simulink model "ROV_Simulation_openloop_ver2"  (R2023a)
settings: Solver=ode15s  StartTime=0.0  StopTime=Sim.ts  FixedStep=0.01  MaxStep=0.01  MinStep=0.0001  RelTol=1e-3
undefined symbols (not defined in the file): ext, hyd, ics, phy, rb, thrust, VC
libraries: simulink_extras x3, simulink x1
settings Model: Creator=dmmavani  LastModifiedBy=dmmavani
settings SolverCC: ConcurrentTasks=on  PositivePriorityOrder=on  AutoInsertRateTranBlk=on
settings DataIOCC: InspectSignalLogs=on
settings OptimizationCC: BlockReduction=off  DefaultParameterBehavior=Inlined  EnhancedBackFolding=on  PassReuseOutputArgsAs=Individual arguments  ZeroExternalMemoryAtStartup=off  ZeroInternalMemoryAtStartup=off  OptimizeBlockOrder=speed  DifferentSizesBufferReuse=on  OptimizationCustomize=off  EfficientTunableParamExpr=on
settings DebuggingCC: TasksWithSamePriorityMsg=none  ParameterTunabilityLossMsg=error
settings HardwareCC: ProdBitPerLong=64  ProdLongLongMode=on  ProdHWDeviceType=Intel->x86-64 (Linux 64)
settings SFSimCC: MATLABDynamicMemAlloc=off
settings RTWCC: Description=Embedded Coder  SystemTargetFile=ert.tlc  GenCodeOnly=on  TemplateMakefile=ert_default_tmf  Toolchain=Simulink Real-Time Toolchain  BuildConfiguration=Faster Runs  CodeExecutionProfiling=on  TargetLang=C++
settings CodeAppCC: ForceParamTrailComments=on  IgnoreCustomStorageClasses=off  OperatorAnnotations=on  SimulinkDataObjDesc=on  SFDataObjDesc=on  InsertBlockDesc=on
settings ERTTargetCC: TargetLangStandard=C++03 (ISO)  GenerateSampleERTMain=on  CodeInterfacePackaging=C++ class  InlinedParameterPlacement=NonHierarchical  RootIOFormat=Structure reference  ERTCustomFileTemplate=example_file_process.tlc

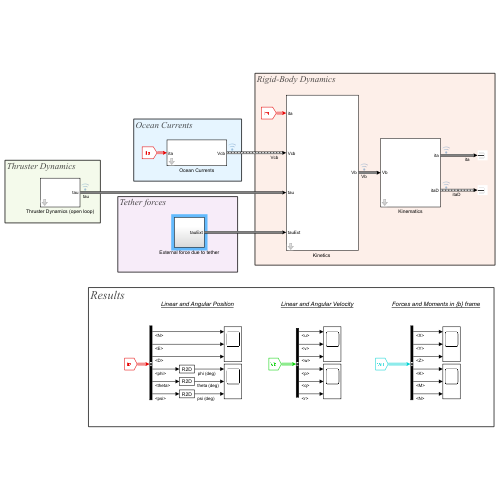
[thumbnail: Simulink's stored preview of the top-level diagram]
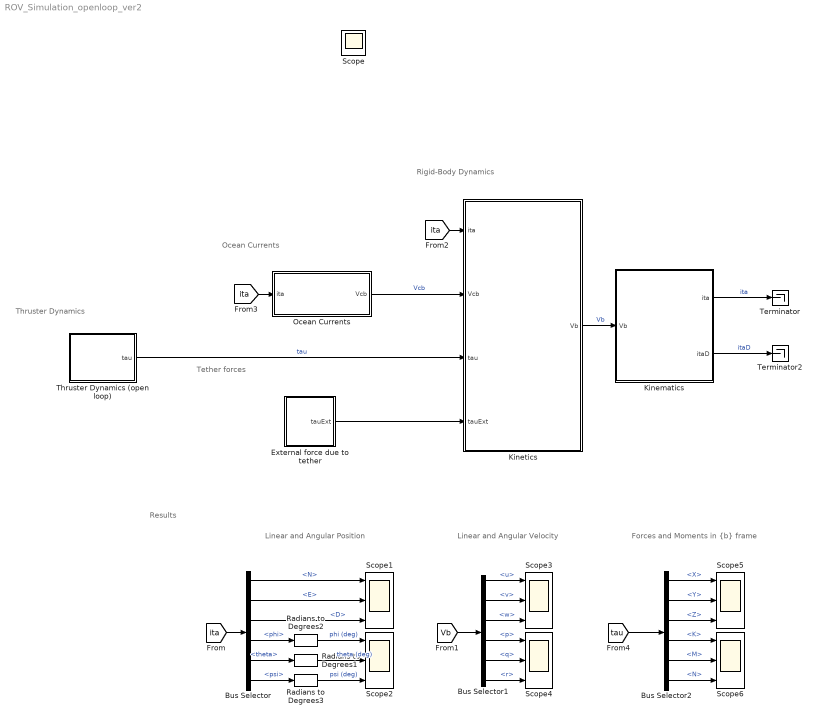
== system ROV_Simulation_openloop_ver2 ==
  note: Results
  note: Linear and Angular Position
  note: Tether forces
  note: Thruster Dynamics
  note: Ocean Currents
  note: Rigid-Body Dynamics
  note: Linear and Angular Velocity
  note: Forces and Moments in {b} frame
  Bus Selector : BusSelector  OutputSignals=N,E,D,phi,theta,psi
  Bus Selector1 : BusSelector  OutputSignals=u,v,w,p,q,r
  Bus Selector2 : BusSelector  OutputSignals=X,Y,Z,K,M,N
  External force due to tether : Subsystem
  Kinematics : Subsystem  mask{Parameter7=|, North=ics.ita.N, East=ics.ita.E, Down=ics.ita.D, Roll=ics.ita.phi, Pitch=ics.ita.theta, InitialCondition=ics.ita.psi}
      mask Parameter7=|
      | Kinematics block is used to transform velocities from BODY to
      | NED frame.
      |
      | itaD = J(euler) * Vb    ( Velocities in NED frame)
      | J(euler) = Transformation Matrix (function of euler angles)
      | Vb = Velocities in BODY frame.
      mask prompts: North "N :"; East "E :"; Down "D :"; Roll "Roll :"; Pitch "Pitch :"; InitialCondition "Yaw :"
      mask TypeOptions North: Integrator/InitialCondition
      mask TypeOptions East: Integrator1/InitialCondition
      mask TypeOptions Down: Integrator3/InitialCondition
      mask TypeOptions Roll: Integrator4/InitialCondition
      mask TypeOptions Pitch: Integrator5/InitialCondition
      mask TypeOptions InitialCondition: Integrator6/InitialCondition
      mask DialogControl Container4 Prompt: Description
      mask DialogControl Container1 Prompt: Initial Conditions for position and orientation in NED frame
      mask DialogControl Container2 Prompt: Position (meters)
      mask DialogControl Container3 Prompt: Orientation (rad)
  "Kinetics " : Subsystem  mask{Parameter7=|, u_b=ics.vb.u, v_b=ics.vb.v, w_b=ics.vb.w, p_b=ics.vb.p, q_b=ics.vb.q, r_b=ics.vb.r}
      mask Parameter7=|
      | Kinetics block is used to solve the 6DOF equations of motion
      | of a ROV in BODY frame.
      | Block outputs V_b (Velocities in BODY frame).
      mask prompts: u_b "u_b :"; v_b "v_b :"; w_b "w_b :"; p_b "p_b :"; q_b "q_b :"; r_b "r_b :"
      mask TypeOptions u_b: Integrator/InitialCondition
      mask TypeOptions v_b: Integrator1/InitialCondition
      mask TypeOptions w_b: Integrator2/InitialCondition
      mask TypeOptions p_b: Integrator3/InitialCondition
      mask TypeOptions q_b: Integrator4/InitialCondition
      mask TypeOptions r_b: Integrator5/InitialCondition
      mask DialogControl Container4 Prompt: Description
      mask DialogControl InitialCondition Prompt: Initial conditions for velocity of body in {b} frame
      mask DialogControl Container2 Prompt: Linear Velocity  (m/s)
      mask DialogControl Container3 Prompt: Angular Velocity (rad/s)
  Ocean Currents : Subsystem  mask{Parameter1=|, Value=VC}
      mask Parameter1=|
      | If the value is equal to 1 then ocean currents is ON.
      | if the value is equal to 0 then ocean currents is OFF.
      mask prompts: Value "Ocean currents (On/Off):"
      mask TypeOptions Value: Constant1/Value
      mask DialogControl Container2 Prompt: Description
  Radians to Degrees1 : simulink_extras/Transformations/Radians to Degrees
  Radians to Degrees2 : simulink_extras/Transformations/Radians to Degrees
  Radians to Degrees3 : simulink_extras/Transformations/Radians to Degrees
  Scope{1..6} (6 alike) : Scope  NumInputPorts=3
  Terminator : Terminator
  Terminator2 : Terminator
  Thruster Dynamics (open loop) : Subsystem  mask{Parameter2=|, Value=1}
      mask Parameter2=|
      | Step input    (Input type = 1)
      | Impulse input (Input type = 0)
      mask prompts: Value "Input type:"
      mask TypeOptions Value: Constant/Value
      mask DialogControl DescGroupVar Prompt: Description
  Scope : Scope
  wires:
  Ocean Currents/1(Vcb) -> "Kinetics "/2(Vcb)  "Vcb"
  [ita] -> Bus Selector/1
  Bus Selector/1 -> Scope1/1  "<N>"
  Bus Selector/2 -> Scope1/2  "<E>"
  Bus Selector/3 -> Scope1/3  "<D>"
  Bus Selector/4 -> Radians to Degrees2/1  "<phi>"
  Radians to Degrees2/1 -> Scope2/1  "phi (deg)"
  Bus Selector/5 -> Radians to Degrees1/1  "<theta>"
  Bus Selector/6 -> Radians to Degrees3/1  "<psi>"
  [Vb] -> Bus Selector1/1
  Bus Selector1/1 -> Scope3/1  "<u>"
  Bus Selector1/2 -> Scope3/2  "<v>"
  Bus Selector1/3 -> Scope3/3  "<w>"
  Bus Selector1/4 -> Scope4/1  "<p>"
  Bus Selector1/5 -> Scope4/2  "<q>"
  Bus Selector1/6 -> Scope4/3  "<r>"
  Kinematics/1(ita) -> Terminator/1  "ita"
  [ita] -> Ocean Currents/1(ita)
  Thruster Dynamics (open loop)/1(tau) -> "Kinetics "/3(tau)  "tau"
  "Kinetics "/1(Vb) -> Kinematics/1(Vb)  "Vb"
  Kinematics/2(itaD) -> Terminator2/1  "itaD"
  [ita] -> "Kinetics "/1(ita)
  [tau] -> Bus Selector2/1
  Bus Selector2/1 -> Scope5/1  "<X>"
  Bus Selector2/2 -> Scope5/2  "<Y>"
  Bus Selector2/3 -> Scope5/3  "<Z>"
  Bus Selector2/4 -> Scope6/1  "<K>"
  Bus Selector2/5 -> Scope6/2  "<M>"
  Bus Selector2/6 -> Scope6/3  "<N>"
  Radians to Degrees1/1 -> Scope2/2  "theta (deg)"
  Radians to Degrees3/1 -> Scope2/3  "psi (deg)"
  External force due to tether/1(tauExt) -> "Kinetics "/4(tauExt)

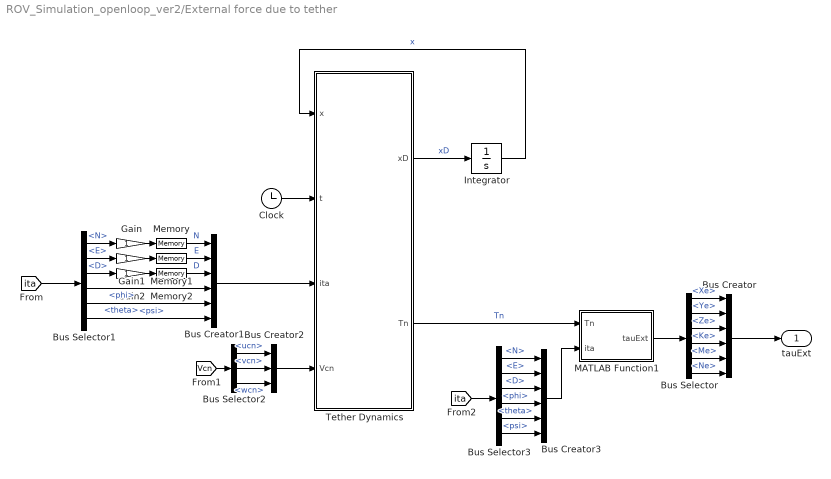
== system ROV_Simulation_openloop_ver2/External force due to tether ==
  Bus Creator : BusCreator  Inputs=6  OutDataTypeStr=Bus: tauExt
  Bus Creator1 : BusCreator  Inputs=6  OutDataTypeStr=Bus: ita
  Bus Creator2 : BusCreator  Inputs=3  OutDataTypeStr=Bus: Vcn
  Bus Creator3 : BusCreator  Inputs=6  OutDataTypeStr=Bus: ita
  Bus Selector : BusSelector  OutputSignals=Xe,Ye,Ze,Ke,Me,Ne
  Bus Selector1 : BusSelector  OutputSignals=N,E,D,phi,theta,psi
  Bus Selector2 : BusSelector  OutputSignals=ucn,vcn,wcn
  Bus Selector3 : BusSelector  OutputSignals=N,E,D,phi,theta,psi
  Clock : Clock
  Gain : Gain
  Gain1 : Gain
  Gain2 : Gain
  Integrator : Integrator  InitialCondition=ics.tether.xstate
  MATLAB Function1 : MATLAB Function  TreatAsAtomicUnit=on
  Memory : Memory  InitialCondition=ics.ita.N
  Memory1 : Memory  InitialCondition=ics.ita.E
  Memory2 : Memory  InitialCondition=ics.ita.D
  Tether Dynamics : MATLAB Function  TreatAsAtomicUnit=on
  tauExt : Outport  OutDataTypeStr=Bus: tauExt
  wires:
  Gain1/1 -> Memory1/1
  Gain2/1 -> Memory2/1
  Bus Selector1/6 -> Bus Creator1/6  "<psi>"
  Memory2/1 -> Bus Creator1/3  "D"
  Memory1/1 -> Bus Creator1/2  "E"
  Bus Creator2/1 -> Tether Dynamics/4(Vcn)
  Tether Dynamics/1(xD) -> Integrator/1  "xD"
  Gain/1 -> Memory/1
  Bus Creator3/1 -> MATLAB Function1/2(ita)
  Bus Selector3/5 -> Bus Creator3/5  "<theta>"
  Bus Selector1/1 -> Gain/1  "<N>"
  Bus Selector2/1 -> Bus Creator2/1  "<ucn>"
  [Vcn] -> Bus Selector2/1
  Clock/1 -> Tether Dynamics/2(t)
  Bus Selector3/4 -> Bus Creator3/4  "<phi>"
  Bus Selector3/1 -> Bus Creator3/1  "<N>"
  Integrator/1 -> Tether Dynamics/1(x)  "x"
  MATLAB Function1/1(tauExt) -> Bus Selector/1
  Bus Selector3/2 -> Bus Creator3/2  "<E>"
  [ita] -> Bus Selector1/1
  Memory/1 -> Bus Creator1/1  "N"
  Bus Selector1/5 -> Bus Creator1/5  "<theta>"
  [ita] -> Bus Selector3/1
  Bus Selector1/4 -> Bus Creator1/4  "<phi>"
  Bus Selector3/3 -> Bus Creator3/3  "<D>"
  Bus Selector1/2 -> Gain1/1  "<E>"
  Tether Dynamics/2(Tn) -> MATLAB Function1/1(Tn)  "Tn"
  Bus Selector/6 -> Bus Creator/6  "<Ne>"
  Bus Selector1/3 -> Gain2/1  "<D>"
  Bus Creator1/1 -> Tether Dynamics/3(ita)
  Bus Selector/4 -> Bus Creator/4  "<Ke>"
  Bus Selector/5 -> Bus Creator/5  "<Me>"
  Bus Selector/3 -> Bus Creator/3  "<Ze>"
  Bus Selector/2 -> Bus Creator/2  "<Ye>"
  Bus Selector2/2 -> Bus Creator2/2  "<vcn>"
  Bus Creator/1 -> tauExt/1
  Bus Selector2/3 -> Bus Creator2/3  "<wcn>"
  Bus Selector/1 -> Bus Creator/1  "<Xe>"
  Bus Selector3/6 -> Bus Creator3/6  "<psi>"

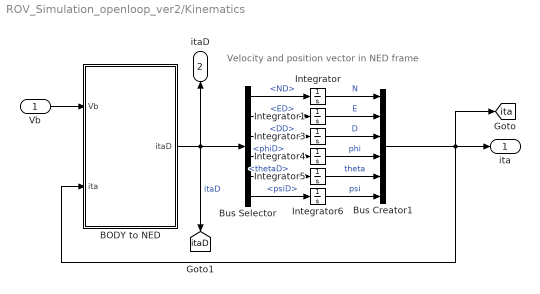
== system ROV_Simulation_openloop_ver2/Kinematics ==
  note: Velocity and position vector in
      |  NED frame
  Vb : Inport  OutDataTypeStr=Bus: Vb
  " BODY to NED" : MATLAB Function  TreatAsAtomicUnit=on
  Bus Creator1 : BusCreator  Inputs=6  OutDataTypeStr=Bus: ita
  Bus Selector : BusSelector  OutputSignals=ND,ED,DD,phiD,thetaD,psiD
  Integrator : Integrator  InitialCondition=North  LowerSaturationLimit=ics.N
  Integrator1 : Integrator  InitialCondition=East  LowerSaturationLimit=ics.E
  Integrator3 : Integrator  InitialCondition=Down  LowerSaturationLimit=ics.D
  Integrator4 : Integrator  InitialCondition=Roll  LowerSaturationLimit=ics.phi
  Integrator5 : Integrator  InitialCondition=Pitch  LowerSaturationLimit=ics.theta
  Integrator6 : Integrator  InitialCondition=InitialCondition  LowerSaturationLimit=ics.psi
  ita : Outport  OutDataTypeStr=Bus: ita
  itaD : Outport  Port=2  OutDataTypeStr=Bus: itaD
  tag scope: ita=global, itaD=global
  wires:
  " BODY to NED"/1(itaD) -> Bus Selector/1, [itaD], itaD/1  "itaD"
  Bus Creator1/1 -> [ita], ita/1, " BODY to NED"/2(ita)
  Bus Selector/1 -> Integrator/1  "<ND>"
  Bus Selector/2 -> Integrator1/1  "<ED>"
  Bus Selector/6 -> Integrator6/1  "<psiD>"
  Bus Selector/5 -> Integrator5/1  "<thetaD>"
  Bus Selector/3 -> Integrator3/1  "<DD>"
  Bus Selector/4 -> Integrator4/1  "<phiD>"
  Integrator/1 -> Bus Creator1/1  "N"
  Integrator1/1 -> Bus Creator1/2  "E"
  Integrator3/1 -> Bus Creator1/3  "D"
  Integrator4/1 -> Bus Creator1/4  "phi"
  Integrator5/1 -> Bus Creator1/5  "theta"
  Integrator6/1 -> Bus Creator1/6  "psi"
  Vb/1 -> " BODY to NED"/1(Vb)

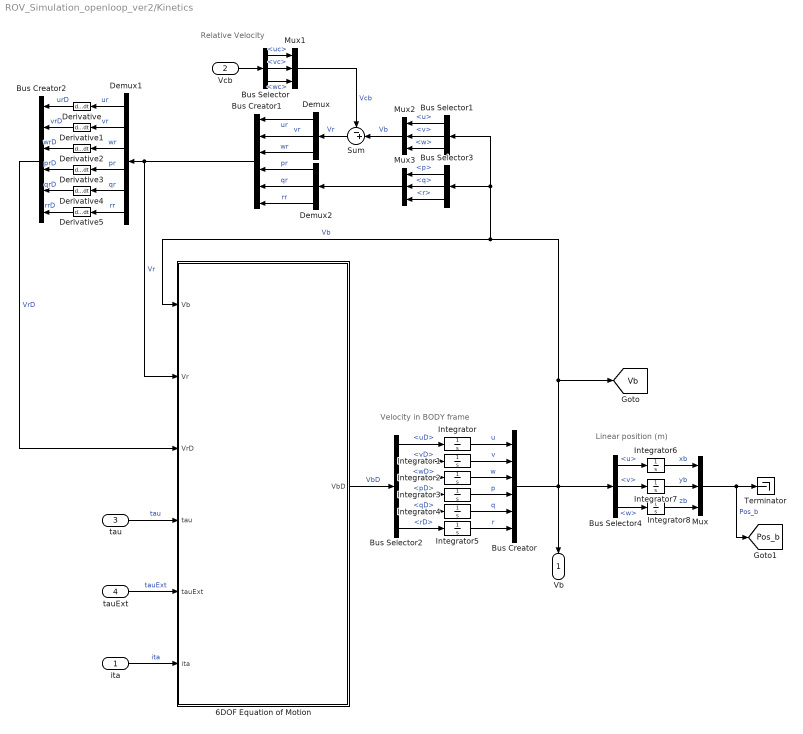
== system ROV_Simulation_openloop_ver2/Kinetics  ==
  note: Linear position (m)
  note: Velocity in BODY frame
  note: Relative Velocity
  ita : Inport  OutDataTypeStr=Bus: ita
  Vcb : Inport  Port=2  OutDataTypeStr=Bus: Vcb
  tau : Inport  Port=3  OutDataTypeStr=Bus: tau
  tauExt : Inport  Port=4  OutDataTypeStr=Bus: tauExt
  "6DOF Equation of Motion " : MATLAB Function  TreatAsAtomicUnit=on
  Bus Creator : BusCreator  Inputs=6  OutDataTypeStr=Bus: Vb
  Bus Creator1 : BusCreator  Inputs=6  OutDataTypeStr=Bus: Vr
  Bus Creator2 : BusCreator  Inputs=6  OutDataTypeStr=Bus: VrD
  Bus Selector : BusSelector  OutputSignals=uc,vc,wc
  Bus Selector1 : BusSelector  OutputSignals=u,v,w
  Bus Selector2 : BusSelector  OutputSignals=uD,vD,wD,pD,qD,rD
  Bus Selector3 : BusSelector  OutputSignals=p,q,r
  Bus Selector4 : BusSelector  OutputSignals=u,v,w
  Demux : Demux  Outputs=3
  Demux1 : Demux  Outputs=6
  Demux2 : Demux  Outputs=3
  Derivative{,1..5} (6 alike) : Derivative
  Integrator : Integrator  InitialCondition=u_b  UpperSaturationLimit=ics.sat.umax  LowerSaturationLimit=0
  Integrator1 : Integrator  InitialCondition=v_b  UpperSaturationLimit=ics.sat.vmax  LowerSaturationLimit=0
  Integrator2 : Integrator  InitialCondition=w_b  UpperSaturationLimit=ics.sat.wmax  LowerSaturationLimit=0
  Integrator3 : Integrator  InitialCondition=p_b  UpperSaturationLimit=ics.sat.pmax  LowerSaturationLimit=0
  Integrator4 : Integrator  InitialCondition=q_b  UpperSaturationLimit=ics.sat.qmax  LowerSaturationLimit=0
  Integrator5 : Integrator  InitialCondition=r_b  UpperSaturationLimit=ics.sat.rmax  LowerSaturationLimit=0
  Integrator6 : Integrator  LowerSaturationLimit=0
  Integrator7 : Integrator  LowerSaturationLimit=0
  Integrator8 : Integrator  LowerSaturationLimit=0
  Mux{,1..3} (4 alike) : Mux  Inputs=3
  Sum : Sum  Inputs=-+|
  Terminator : Terminator
  Vb : Outport  OutDataTypeStr=Bus: Vb
  tag scope: Pos_b=global, Vb=global
  wires:
  Mux1/1 -> Sum/1  "Vcb"
  Bus Selector1/1 -> Mux2/1  "<u>"
  Bus Selector1/2 -> Mux2/2  "<v>"
  Bus Selector1/3 -> Mux2/3  "<w>"
  Mux2/1 -> Sum/2  "Vb"
  Bus Creator/1 -> Bus Selector1/1, Bus Selector3/1, "6DOF Equation of Motion "/1(Vb), [Vb], Vb/1, Bus Selector4/1  "Vb"
  ita/1 -> "6DOF Equation of Motion "/6(ita)  "ita"
  tau/1 -> "6DOF Equation of Motion "/4(tau)  "tau"
  "6DOF Equation of Motion "/1(VbD) -> Bus Selector2/1  "VbD"
  Bus Selector2/1 -> Integrator/1  "<uD>"
  Bus Selector2/2 -> Integrator1/1  "<vD>"
  Bus Selector2/3 -> Integrator2/1  "<wD>"
  Bus Selector2/4 -> Integrator3/1  "<pD>"
  Bus Selector2/5 -> Integrator4/1  "<qD>"
  Bus Selector2/6 -> Integrator5/1  "<rD>"
  Vcb/1 -> Bus Selector/1
  Bus Selector/1 -> Mux1/1  "<uc>"
  Bus Selector/2 -> Mux1/2  "<vc>"
  Bus Selector/3 -> Mux1/3  "<wc>"
  Sum/1 -> Demux/1  "Vr"
  Demux/1 -> Bus Creator1/1  "ur"
  Demux/3 -> Bus Creator1/3  "wr"
  Mux3/1 -> Demux2/1
  Demux/2 -> Bus Creator1/2  "vr"
  Demux2/1 -> Bus Creator1/4  "pr"
  Demux2/2 -> Bus Creator1/5  "qr"
  Demux2/3 -> Bus Creator1/6  "rr"
  Integrator/1 -> Bus Creator/1  "u"
  Integrator1/1 -> Bus Creator/2  "v"
  Integrator2/1 -> Bus Creator/3  "w"
  Integrator3/1 -> Bus Creator/4  "p"
  Integrator4/1 -> Bus Creator/5  "q"
  Integrator5/1 -> Bus Creator/6  "r"
  Bus Selector3/2 -> Mux3/2  "<q>"
  Bus Selector3/3 -> Mux3/3  "<r>"
  Bus Selector3/1 -> Mux3/1  "<p>"
  Bus Selector4/1 -> Integrator6/1  "<u>"
  Bus Selector4/2 -> Integrator7/1  "<v>"
  Bus Selector4/3 -> Integrator8/1  "<w>"
  Integrator6/1 -> Mux/1  "xb"
  Integrator7/1 -> Mux/2  "yb"
  Integrator8/1 -> Mux/3  "zb"
  Mux/1 -> [Pos_b], Terminator/1  "Pos_b"
  Bus Creator1/1 -> Demux1/1, "6DOF Equation of Motion "/2(Vr)  "Vr"
  Demux1/1 -> Derivative/1  "ur"
  Derivative/1 -> Bus Creator2/1  "urD"
  Demux1/2 -> Derivative1/1  "vr"
  Derivative1/1 -> Bus Creator2/2  "vrD"
  Demux1/3 -> Derivative2/1  "wr"
  Derivative2/1 -> Bus Creator2/3  "wrD"
  Demux1/4 -> Derivative3/1  "pr"
  Derivative3/1 -> Bus Creator2/4  "prD"
  Demux1/5 -> Derivative4/1  "qr"
  Derivative4/1 -> Bus Creator2/5  "qrD"
  Demux1/6 -> Derivative5/1  "rr"
  Derivative5/1 -> Bus Creator2/6  "rrD"
  Bus Creator2/1 -> "6DOF Equation of Motion "/3(VrD)  "VrD"
  tauExt/1 -> "6DOF Equation of Motion "/5(tauExt)  "tauExt"

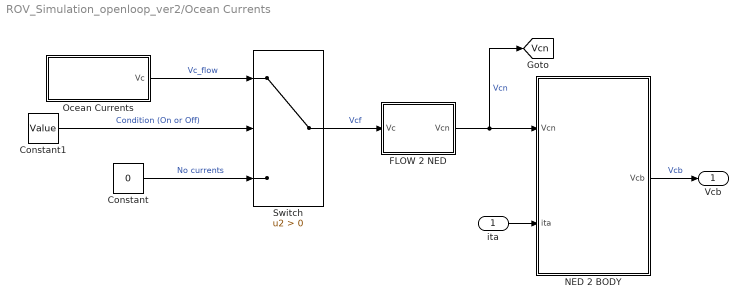
== system ROV_Simulation_openloop_ver2/Ocean Currents ==
  ita : Inport  OutDataTypeStr=Bus: ita
  Constant : Constant  Value=0
  Constant1 : Constant  Value=Value
  FLOW 2 NED : MATLAB Function  TreatAsAtomicUnit=on
  NED 2 BODY : MATLAB Function  TreatAsAtomicUnit=on
  Ocean Currents : Subsystem  Variant=on
  Switch : Switch  Criteria=u2 > Threshold  SaturateOnIntegerOverflow=off  InputSameDT=off
  Vcb : Outport  OutDataTypeStr=Bus: Vcb
  tag scope: Vcn=global
  wires:
  Ocean Currents/1(Vc) -> Switch/1  "Vc_flow"
  Constant/1 -> Switch/3  "No currents"
  Switch/1 -> FLOW 2 NED/1(Vc)  "Vcf"
  Constant1/1 -> Switch/2  "Condition (On or Off)"
  FLOW 2 NED/1(Vcn) -> NED 2 BODY/1(Vcn), [Vcn]  "Vcn"
  ita/1 -> NED 2 BODY/2(ita)
  NED 2 BODY/1(Vcb) -> Vcb/1  "Vcb"

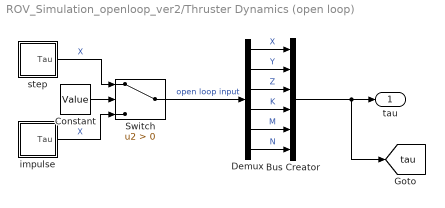
== system ROV_Simulation_openloop_ver2/Thruster Dynamics (open loop) ==
  Bus Creator : BusCreator  Inputs=6  OutDataTypeStr=Bus: tau
  Constant : Constant  Value=Value
  Demux : Demux  Outputs=6
  Switch : Switch  Criteria=u2 > Threshold  SaturateOnIntegerOverflow=off  InputSameDT=off
  impulse : Subsystem
  step : Subsystem
  tau : Outport  OutDataTypeStr=Bus: tau
  tag scope: tau=global
  wires:
  Demux/2 -> Bus Creator/2  "Y"
  Demux/3 -> Bus Creator/3  "Z"
  Demux/4 -> Bus Creator/4  "K"
  Demux/5 -> Bus Creator/5  "M"
  Demux/6 -> Bus Creator/6  "N"
  Bus Creator/1 -> [tau], tau/1
  Demux/1 -> Bus Creator/1  "X"
  step/1(Tau) -> Switch/1  "X"
  impulse/1(Tau) -> Switch/3  "X"
  Constant/1 -> Switch/2
  Switch/1 -> Demux/1  "open loop input"

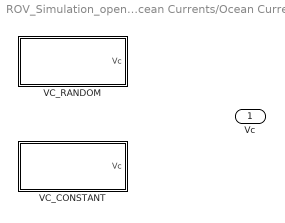
== system ROV_Simulation_openloop_ver2/Ocean Currents/Ocean Currents ==
  VC_CONSTANT : Subsystem  VariantControl=VC_CONSTANT
  VC_RANDOM : Subsystem  VariantControl=VC_RANDOM
  Vc : Outport

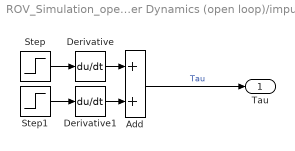
== system ROV_Simulation_openloop_ver2/Thruster Dynamics (open loop)/impulse ==
  Add : Sum
  Derivative : Derivative
  Derivative1 : Derivative
  Step : Step  Time=thrust.start  Before=-thrust.control.Tau  After=-thrust.control.Tau+thrust.control.Tau  SampleTime=0
  Step1 : Step  Time=thrust.start + thrust.duration  Before=thrust.control.Tau  After=0  SampleTime=0
  Tau : Outport
  wires:
  Add/1 -> Tau/1  "Tau"
  Step/1 -> Derivative/1
  Derivative/1 -> Add/1
  Step1/1 -> Derivative1/1
  Derivative1/1 -> Add/2

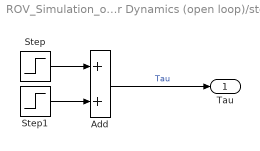
== system ROV_Simulation_openloop_ver2/Thruster Dynamics (open loop)/step ==
  Add : Sum
  Step : Step  Time=thrust.start  Before=-thrust.control.Tau  After=-thrust.control.Tau+thrust.control.Tau  SampleTime=0
  Step1 : Step  Time=thrust.duration+thrust.start  Before=thrust.control.Tau  After=0  SampleTime=0
  Tau : Outport
  wires:
  Step1/1 -> Add/2
  Step/1 -> Add/1
  Add/1 -> Tau/1  "Tau"

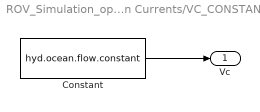
== system ROV_Simulation_openloop_ver2/Ocean Currents/Ocean Currents/VC_CONSTANT ==
  Constant : Constant  Value=hyd.ocean.flow.constant
  Vc : Outport
  wires:
  Constant/1 -> Vc/1

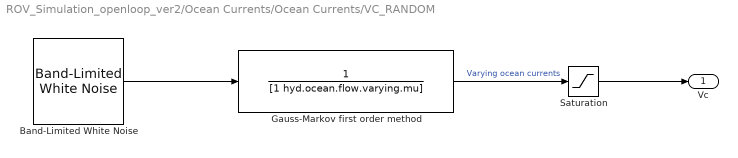
== system ROV_Simulation_openloop_ver2/Ocean Currents/Ocean Currents/VC_RANDOM ==
  Band-Limited White Noise : simulink/Sources/Band-Limited White Noise  Cov=hyd.ocean.flow.noise.power  Ts=hyd.ocean.flow.noise.ts  seed=[23341]
  Gauss-Markov first order method : TransferFcn  Denominator=[1 hyd.ocean.flow.varying.mu]
  Saturation : Saturate  UpperLimit=hyd.ocean.flow.varying.Vmax  LowerLimit=hyd.ocean.flow.varying.Vmin
  Vc : Outport
  wires:
  Band-Limited White Noise/1 -> Gauss-Markov first order method/1
  Gauss-Markov first order method/1 -> Saturation/1  "Varying ocean currents"
  Saturation/1 -> Vc/1

== matlab function ROV_Simulation_openloop_ver2/Kinematics/ BODY to NED ==
  data: itaD output Bus: itaD size=1; Vb input Bus: Vb size=1; ita input Bus: ita
function itaD = Vn(Vb,ita)

vb = [Vb.u,Vb.v,Vb.w,Vb.p,Vb.q,Vb.r]';

% Euler angles
phi = ita.phi;
theta = ita.theta;
psi = ita.psi;

% Rotational matrices (Linear & angular)
Rbn = rotbn(phi,theta,psi);
Tbn = tbn(phi,theta);

% J is transformation matrix
J = [Rbn,zeros(3);zeros(3),Tbn];

% if t>40
%     a=3;
% end

z = J*vb;       % Transformation of velocity from {b} to {n} frame

% Velocity of ROV in NED / {n} frame 
itaD.ND = z(1);
itaD.ED = z(2);
itaD.DD = z(3);
itaD.phiD = z(4);
itaD.thetaD = z(5);
itaD.psiD = z(6);

== matlab function ROV_Simulation_openloop_ver2/Ocean Currents/FLOW 2 NED ==
  data: Vc input; Vcn output Bus: Vcn; hyd parameter
function Vcn = f2e(Vc,hyd)

Rfn = R_alpha(hyd)'*R_beta(hyd)';

xx = Rfn * [Vc,0,0]';        % Velocity vector in {n} frame

% Ocean current in NED / {n} frame
Vcn.ucn = xx(1);
Vcn.vcn = xx(2);
Vcn.wcn = xx(3);

== matlab function ROV_Simulation_openloop_ver2/Kinetics /6DOF Equation of Motion  ==
  data: Vb input Bus: Vb size=1; Vr input Bus: Vr size=1; VrD input Bus: VrD; tau input Bus: tau size=1; VbD output Bus: VbD size=1; tauExt input Bus: tauExt; ita input Bus: ita size=1; rb parameter; hyd parameter; phy parameter
function VbD = eomRB(Vb, Vr, VrD, tau, tauExt, ita, rb, hyd, phy)

% Equation of motion or kinetic equation can be derived using Mrb (Mass
% matrix), Crb (Coriolis-Centripetal force) and vb (velocity of vehicle in
% body-fixed frame {b}
% EOM is Mrb*vDot + Crb(vb)*vb = tau_RB       


vb = [Vb.u,Vb.v,Vb.w,Vb.p,Vb.q,Vb.r]';
vr = [Vr.ur,Vr.vr,Vr.wr,Vr.pr,Vr.qr,Vr.rr]';
vrd = [VrD.urD, VrD.vrD, VrD.wrD, VrD.prD, VrD.qrD, VrD.rrD]';
Tau = [tau.X,tau.Y,tau.Z,tau.K,tau.M,tau.N]';
tauExt = [tauExt.Xe,tauExt.Ye,tauExt.Ze,tauExt.Ke,tauExt.Me,tauExt.Ne]';
MRB = Mrb(rb);
CRB = Crb(rb,Vb);
MA = Ma(hyd);
CA = Ca(hyd,Vr);
Dl = DL(hyd);
Dnl = DNL(hyd,Vr);
g_ita = hydStat(ita,rb,phy,hyd);


y = (-(CRB*vb) - MA*vrd - (CA*vr) - ((Dl+Dnl)*vr) - g_ita + Tau + tauExt)./(MRB*ones(6,1));

% Velocity in BODY or {b} frame
VbD.uD = y(1);
VbD.vD = y(2);
VbD.wD = y(3);
VbD.pD = y(4);
VbD.qD = y(5);
VbD.rD = y(6);

== matlab function ROV_Simulation_openloop_ver2/Ocean Currents/NED 2 BODY ==
  data: Vcn input Bus: Vcn; ita input Bus: ita; Vcb output Bus: Vcb
function Vcb = e2b(Vcn,ita)

% Rotation matrix 
Rbn = rotbn(ita.phi,ita.theta,ita.psi);
x = [Vcn.ucn;Vcn.vcn;Vcn.wcn];
tmp = Rbn' * x;       

% Velocity of currents in {b} frame
Vcb.uc = tmp(1);
Vcb.vc = tmp(2);
Vcb.wc = tmp(3);

== matlab function ROV_Simulation_openloop_ver2/External force due to tether/Tether Dynamics ==
  data: x input; t input; ita input Bus: ita; Vcn input Bus: Vcn; xD output; Tn output; ext parameter; phy parameter
function [xD,Tn] = pDD(x,t,ita,Vcn, ext,phy)
% Input by the user
%%%%%%%%%%%%%%%%%%%%%%%%%%%%%%%%%%%%%%%%%%%%%%%%%%%%
n = 9;         % no of nodes ---- (total nodes - 2)
%%%%%%%%%%%%%%%%%%%%%%%%%%%%%%%%%%%%%%%%%%%%%%%%%%%%

 if t == 4
    a = 3;
 end
E = ext.tether.E;
m = ext.tether.m;
l0 = ext.tether.init.lu;
rho = phy.rho;
Cint = ext.tether.Cint;
Cn = ext.tether.Cn;
Ct = ext.tether.Ct;
dt = ext.tether.d;

xState = x;
xstate = reshape(xState,3,[]);
% let define state vector
    p0 = ext.tether.init.r0;      % position of first node
    pn = [ita.N,ita.E,ita.D]';     % position of last node (attached to ROV)
    pr = xstate(:,1:n);      % position of remaining nodes 
    v0 = zeros(3,1);
    vr = xstate(:,n+1:2*n);
    vc = [Vcn.ucn,Vcn.vcn,Vcn.wcn]';
   

% Mass matrix
M = (((m*l0)) + (pi/4)*dt.^2*l0*rho) * ones(3,1); 
%% Internal forces
    % Tension in N-2 nodes  
        K = (E*(pi/4)*dt^2)/l0;
        T = zeros(3,n);
        for i = 1:n
            if i<n
                % ab = l0/norm(pr(:,i+1) - pr(:,i));
                % if abs(1 - ab) < 1e-6
                %     ab = 1;
                % else
                %     % do nothing
                % end
                T(:,i) = K * (pr(:,i+1)-pr(:,i)) * (1-(l0/norm(pr(:,i+1) - pr(:,i))));
            elseif i==n
                % bc = l0/norm(pn - pr(:,i));
                % if abs(1 - bc) < 1e-6
                %     bc = 1;
                % else
                %     % do nothing
                % end
                T(:,i) = K * (pn - pr(:,i)) * (1-(l0/norm(pn - pr(:,i))));
            end
        end
       
        T1 = K * (pr(:,1)-p0) * (1-(l0/norm(pr(:,1)-p0)));

    % Internal damping
        Pi = zeros(3,n);      % Internal Damping
        for i = 1:n
            if i==1
                Pi(:,i) = (Cint/l0)*((vr(:,i) - v0)' * (pr(:,i+1)-pr(:,i))) * ((pr(:,i+1)-pr(:,i))./norm(pr(:,i+1)-pr(:,i))^2) ;
            elseif (i>1)&&(i<n)
                Pi(:,i) = (Cint/l0)*((vr(:,i) - vr(:,i-1))' * (pr(:,i+1)-pr(:,i))) * ((pr(:,i)-pr(:,i+1))./norm(pr(:,i)-pr(:,i+1))^2);
            elseif i == n
                Pi(:,i) = (Cint/l0)*((vr(:,i) - vr(:,i-1))' * (pn - pr(:,i))) * ((pn - pr(:,i))./norm(pn - pr(:,i))^2);
            end
        end
        P1 = ((Cint/l0) * ((v0)' * (pr(:,1) - p0))) * ((pr(:,1) - p0)./norm(pr(:,1) - p0)^2);
    
%% External forces
    % Hydrodynamic force/Damping
            % Normal and Tangential velocity component
                 Vt = zeros(3,n);
                for i = 1:n
                    if i<n
                        Vt(:,i) = ((vc - vr(:,i))'* (pr(:,i+1)-pr(:,i))) * ((pr(:,i+1)-pr(:,i))./norm(pr(:,i+1)-pr(:,i))^2);
                    elseif i==n
                        Vt(:,i) = ((vc - vr(:,i))'* (pn - pr(:,i))) * ((pn - pr(:,i))./norm(pn - pr(:,i))^2);
                    end
                end
        
                Vn = zeros(3,n);
                for i = 1:n
                    Vn(:,i) = vc - Vt(:,i);
                end
            
               
            % Normal and tangential force component
                Fn = zeros(3,n);
                for i =1:n
                    if i<n
                        Fn(:,i) = 0.5*rho*dt*Cn* Vn(:,i).* abs(Vn(:,i))* norm(pr(:,i+1)-pr(:,i));
                    else
                        Fn(:,i) = 0.5*rho*dt*Cn* Vn(:,i).* abs(Vn(:,i))* norm(pn - pr(:,i));
                    end
                end
            
                Ft = zeros(3,n);
                for i =1:n
                    if i<n
                        Ft(:,i) = 0.5*rho*dt*Ct* Vt(:,i).* abs(Vt(:,i))* norm(pr(:,i+1)-pr(:,i));
                    else
                        Ft(:,i) = 0.5*rho*dt*Ct* Vt(:,i).* abs(Vt(:,i))* norm(pn - pr(:,i));
                    end
                end
        
            % Total hydrodynamic forces
                F = zeros(3,n);
                for i = 1:n
                    F(:,i) = (Fn(:,i) + Ft(:,i));
                end 
            

%% Equation of motion
    vd = zeros(3,n);
    for i=1:n
        if i==1
            vd(:,i) = ((T(:,i) - T1) + (Pi(:,i) - P1) + F(:,i))./M;
        elseif i>1
            vd(:,i) = ((T(:,i) - T(:,i-1)) + (Pi(:,i) - Pi(:,i-1)) + F(:,i))./M;
        end
    end
   
    xD = [reshape(vr,[],1);reshape(vd,[],1)];
    Tn = T(:,end);
 
   
end

== matlab function ROV_Simulation_openloop_ver2/External force due to tether/MATLAB Function1 ==
  data: Tn input; tauExt output Bus: tauExt; ita input
function tauExt = fcn(Tn,ita)

Rbn = rotbn(ita.phi,ita.theta,ita.psi);
Tbn = tbn(ita.phi,ita.theta);
y = [Rbn', zeros(3);zeros(3),Tbn']*[Tn;zeros(3,1)];

% Tether forces and moments
tauExt.Xe = y(1);
tauExt.Ye = y(2);
tauExt.Ze = y(3);
tauExt.Ke = y(4);
tauExt.Me = y(5);
tauExt.Ne = y(6);
